simulink model "filter"  (R2023b)
settings: Solver=VariableStepAuto  StartTime=0.0  StopTime=10000  RelTol=1e-3
settings Model: Creator=user  LastModifiedBy=user

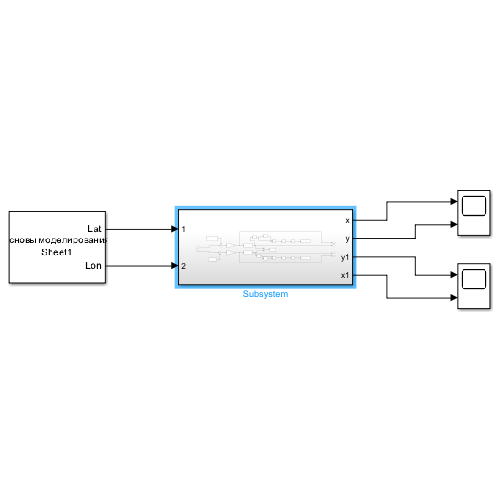
[thumbnail: Simulink's stored preview of the top-level diagram]
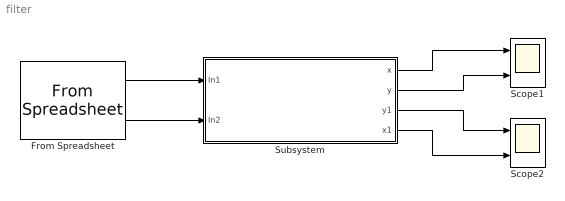
== system filter ==
  From Spreadsheet : FromSpreadsheet  FileName=C:\Users\user\Desktop\Antonov\основы моделирования\3 занятие\LatLon\LatLon1.xlsx
  Scope1 : Scope  NumInputPorts=2
  Scope2 : Scope  NumInputPorts=2
  Subsystem : Subsystem
  wires:
  From Spreadsheet/1 -> Subsystem/1(In1)
  From Spreadsheet/2 -> Subsystem/2(In2)
  Subsystem/1(x) -> Scope1/1
  Subsystem/2(y) -> Scope1/2
  Subsystem/3(y1) -> Scope2/1
  Subsystem/4(x1) -> Scope2/2

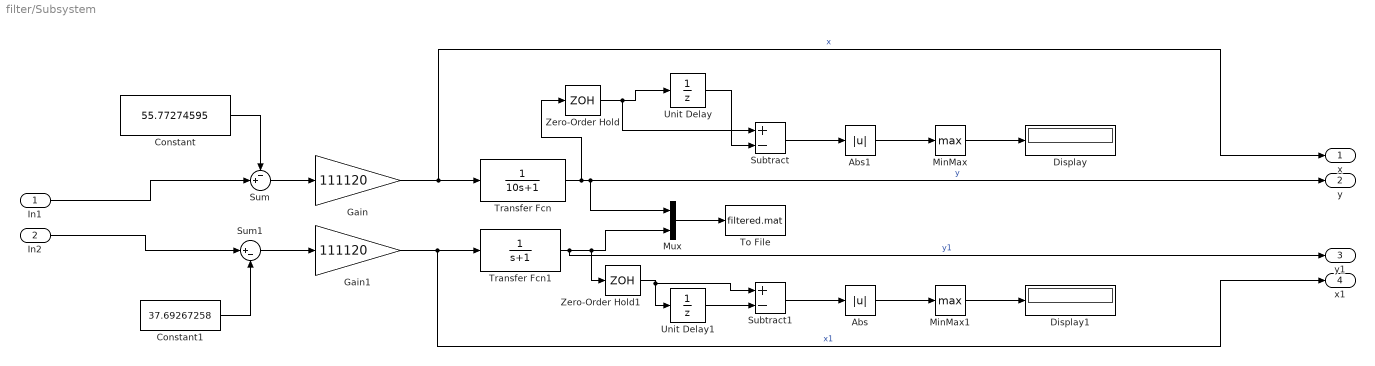
== system filter/Subsystem ==
  In1 : Inport
  In2 : Inport  Port=2
  Abs : Abs  SaturateOnIntegerOverflow=off
  Abs1 : Abs  SaturateOnIntegerOverflow=off
  Constant : Constant  Value=55.77274595
  Constant1 : Constant  Value=37.69267258
  Display : Display
  Display1 : Display
  Gain : Gain  Gain=111120
  Gain1 : Gain  Gain=111120
  MinMax : MinMax  Function=max
  MinMax1 : MinMax  Function=max
  Mux : Mux  Inputs=2
  Subtract : Sum  Inputs=+-
  Subtract1 : Sum  Inputs=+-
  Sum : Sum  Inputs=-+|
  Sum1 : Sum  Inputs=|+-
  To File : ToFile  Filename=filtered.mat  MatrixName=simout
  Transfer Fcn : TransferFcn  Denominator=[10 1]
  Transfer Fcn1 : TransferFcn  Denominator=[1 1]
  Unit Delay : UnitDelay  SampleTime=-1  HasFrameUpgradeWarning=on
  Unit Delay1 : UnitDelay  SampleTime=-1  HasFrameUpgradeWarning=on
  Zero-Order Hold : ZeroOrderHold
  Zero-Order Hold1 : ZeroOrderHold
  x : Outport
  y : Outport  Port=2
  y1 : Outport  Port=3
  x1 : Outport  Port=4
  wires:
  Zero-Order Hold1/1 -> Subtract1/1, Unit Delay1/1
  Subtract/1 -> Abs1/1
  Subtract1/1 -> Abs/1
  Unit Delay1/1 -> Subtract1/2
  MinMax/1 -> Display/1
  Sum/1 -> Gain/1
  Abs/1 -> MinMax1/1
  Transfer Fcn1/1 -> y1/1, Zero-Order Hold1/1, Mux/2  "y1"
  Gain/1 -> x/1, Transfer Fcn/1  "x"
  Gain1/1 -> x1/1, Transfer Fcn1/1  "x1"
  Mux/1 -> To File/1
  Abs1/1 -> MinMax/1
  MinMax1/1 -> Display1/1
  Transfer Fcn/1 -> Zero-Order Hold/1, y/1, Mux/1  "y"
  Constant/1 -> Sum/1
  Unit Delay/1 -> Subtract/2
  Constant1/1 -> Sum1/2
  Zero-Order Hold/1 -> Subtract/1, Unit Delay/1
  Sum1/1 -> Gain1/1
  In2/1 -> Sum1/1
  In1/1 -> Sum/2
